simulink model "FOC_Motor_Control"  (R2020b)
settings: Solver=FixedStepDiscrete  StartTime=0.0  StopTime=10.0  FixedStep=Fixed_Step_Size  RelTol=1e-3
values from neighbouring files (symbols this model uses):
  Angle = 1.0    [Hall_Flux_FOC_Data.sldd]    (also in Motor_Control_Data.sldd)
  Cosine_table = 1.0 0.99999529 0.99999058 0.99998587 0.99998116 0.99996704 0.99995291 0.99993885 0.99992472 0.99990118 0.99987763 0.99985409 0.9998306 0.99979764 0.99976468 0.99973178 0.99969882 0.99965644 0.99961412 0.99957174 0.99952942 0.99947762 0.99942589 0.99937415 0.99932235 0.9992612 0.99920005 0.99913889 0.99907768 0.99900717 0.99893659 0.99886602 0.99879545 0.99871546 0.99863547 0.99855554 0.99847555 0.    [Hall_Flux_FOC_Data.sldd]    (also in Motor_Control_Data.sldd)
  Flux = 0.0109    [G474_FOC_LADRC.sldd]    (also in G474_FOC_NONOBSERVER.sldd = 0.0109
  HaLL_AngleShift = -0.25    [Hall_Flux_FOC_Data.sldd]
  HaLL_Sector1 = 5.236    [Hall_Flux_FOC_Data.sldd]
  HaLL_Sector2 = 1.0472    [Hall_Flux_FOC_Data.sldd]
  HaLL_Sector3 = 0.0    [Hall_Flux_FOC_Data.sldd]
  HaLL_Sector4 = 3.1415    [Hall_Flux_FOC_Data.sldd]
  HaLL_Sector5 = 4.1888    [Hall_Flux_FOC_Data.sldd]
  HaLL_Sector6 = 2.0944    [Hall_Flux_FOC_Data.sldd]
  HaLL_Timer_T = 1.0E-5    [Hall_Flux_FOC_Data.sldd]
  ID_Ki = 1.3    [Hall_Flux_FOC_Data.sldd]    (also in Motor_Control_Data.sldd = 48.0
  ID_Kp = 0.4    [Hall_Flux_FOC_Data.sldd]    (also in Motor_Control_Data.sldd = 0.84
  inverter = struct    [PMSM_Parameters.m]
  IQ_Ki = 1.6    [Hall_Flux_FOC_Data.sldd]    (also in Motor_Control_Data.sldd = 48.0
  IQ_Kp = 0.4    [Hall_Flux_FOC_Data.sldd]    (also in Motor_Control_Data.sldd = 1.869
  LADRC_b0 = 10000.0    [G474_FOC_LADRC.sldd]    (also in Hall_Flux_FOC_Data.sldd = 80000.0
  LADRC_Omega_c = 100.0    [G474_FOC_LADRC.sldd]    (also in Hall_Flux_FOC_Data.sldd = 80.0
  Ld = 0.0004    [Hall_Flux_FOC_Data.sldd]    (also in Motor_Control_Data.sldd = 0.00014
  Lq = 0.00045    [Hall_Flux_FOC_Data.sldd]    (also in Motor_Control_Data.sldd = 0.0003115
  OPL_Speed = 800.0    [Hall_Flux_FOC_Data.sldd]
  OPL_Time = 2.0    [Hall_Flux_FOC_Data.sldd]
  OPL_Torque = 3.0    [Hall_Flux_FOC_Data.sldd]
  Over_modulation = 0.0    [Hall_Flux_FOC_Data.sldd]    (also in Motor_Control_Data.sldd)
  pll_omega = 5000.0    [G474_FOC_LADRC.sldd]    (also in G474_FOC_NONOBSERVER.sldd)
  pll_xi = 10.0    [G474_FOC_LADRC.sldd]    (also in G474_FOC_NONOBSERVER.sldd)
  Pole_Pairs = 2.0    [Hall_Flux_FOC_Data.sldd]    (also in Motor_Control_Data.sldd = 4.0
  PWM_Frequency = 10000.0    [Hall_Flux_FOC_Data.sldd]    (also in Motor_Control_Data.sldd = 20000.0
  R = 0.405    [Hall_Flux_FOC_Data.sldd]    (also in Motor_Control_Data.sldd = 0.016
  Sine_table = 0.0 0.0015339879 0.0030679768 0.0046019657 0.0061359555 0.0076698866 0.0092038177 0.010737749 0.012271681 0.013805497 0.015339312 0.016873131 0.018406944 0.019940587 0.021474229 0.023007872 0.024541514 0.026074925 0.027608337 0.029141748 0.03067516 0.032208283 0.033741407 0.035274528 0.036807653 0.038340431 0.039873205 0.04140598 0.042938754 0.04447113 0.046003502 0.047535874 0.049068246 0.0506001    [Hall_Flux_FOC_Data.sldd]    (also in Motor_Control_Data.sldd)
  Speed_Ki = 0.06    [Hall_Flux_FOC_Data.sldd]    (also in Motor_Control_Data.sldd = 10.809
  Speed_Kp = 0.002    [Hall_Flux_FOC_Data.sldd]    (also in Motor_Control_Data.sldd = 0.08
  Speed_PI_OutputMax = 3.0    [Hall_Flux_FOC_Data.sldd]    (also in Motor_Control_Data.sldd = 700.0
  Speed_PI_OutputMin = -5.0    [Hall_Flux_FOC_Data.sldd]    (also in Motor_Control_Data.sldd = -700.0
  SpeedFilter_Fn = 0.3    [Hall_Flux_FOC_Data.sldd]    (also in Motor_Control_Data.sldd = 0.2
  TorqueMode = 0.0    [Hall_Flux_FOC_Data.sldd]    (also in Motor_Control_Data.sldd)
undefined symbols (not defined in the file or in its folder): DiscIntNeverNeededParam, Flux_Gain, Flux_Theta_Enable, magnitude, SVPWM
libraries: simulink x6, dspstat3 x1, pid_lib x1
(part 3 of 3)

== system FOC_Motor_Control/Motor_Control/Motor_Control_Function/Control_Command_2ms/Control_Command_2ms/Speed_PI/Speed_PI/Speed_Control ==
  Err : Inport
  Reset : Inport  Port=2
  Add : Sum
  Cons : Constant  Value=0  OutDataTypeStr=single
  Discrete-Time Integrator : DiscreteIntegrator  ExternalReset=level  SampleTime=-1  ICPrevOutput=DiscIntNeverNeededParam  ICPrevScaledInput=DiscIntNeverNeededParam
  Ki : Constant  Value=Speed_Ki  OutDataTypeStr=single
  Kp : Constant  Value=Speed_Kp  OutDataTypeStr=single
  Product : Product
  Product1 : Product
  Relational Operator1 : RelationalOperator  Operator===  OutDataTypeStr=boolean  RndMeth=Simplest
  Saturation : Saturate  UpperLimit=Speed_PI_OutputMax  LowerLimit=Speed_PI_OutputMin
  Scope : Scope
  Switch : Switch  Criteria=u2 > Threshold
  Unit Delay3 : UnitDelay  SampleTime=-1  HasFrameUpgradeWarning=on
  PI_Out : Outport
  wires:
  Kp/1 -> Product/1
  Err/1 -> Switch/1, Product/2
  Switch/1 -> Product1/2
  Product1/1 -> Discrete-Time Integrator/1
  Product/1 -> Add/1
  Add/1 -> Relational Operator1/1, Saturation/1
  Saturation/1 -> Relational Operator1/2, PI_Out/1
  Discrete-Time Integrator/1 -> Add/2, Scope/1
  Relational Operator1/1 -> Unit Delay3/1
  Ki/1 -> Product1/1
  Unit Delay3/1 -> Switch/2
  Cons/1 -> Switch/3
  Reset/1 -> Discrete-Time Integrator/2

== system FOC_Motor_Control/Motor_Control/Motor_Control_Function/FOC_Control_100us/FOC/D_Current_PI/ID_Control/Normal ==
  Bus_voltage : Inport
  Action Port : ActionPort  ActionPortLabel=elseif(u1==0)
  Gain : Gain  Gain=1/sqrt(3)
  Gain1 : Gain  Gain=-1/sqrt(3)
  Out1 : Outport
  Out2 : Outport  Port=2
  wires:
  Bus_voltage/1 -> Gain1/1, Gain/1
  Gain/1 -> Out1/1
  Gain1/1 -> Out2/1

== system FOC_Motor_Control/Motor_Control/Motor_Control_Function/FOC_Control_100us/FOC/D_Current_PI/ID_Control/Over_M ==
  Bus_voltage : Inport
  Action Port : ActionPort  ActionPortLabel=if(u1==1)
  Gain : Gain  Gain=2/3
  Gain1 : Gain  Gain=-2/3
  Out1 : Outport
  Out2 : Outport  Port=2
  wires:
  Bus_voltage/1 -> Gain1/1, Gain/1
  Gain/1 -> Out1/1
  Gain1/1 -> Out2/1

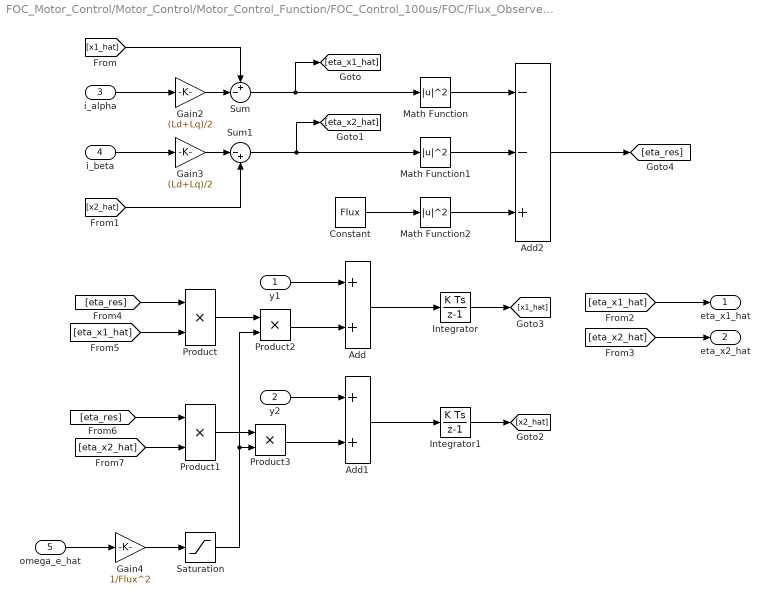
== system FOC_Motor_Control/Motor_Control/Motor_Control_Function/FOC_Control_100us/FOC/Flux_Observer/OBSERVER/Cacl_X1X2_Hat ==
  y1 : Inport  OutDataTypeStr=single
  y2 : Inport  Port=2  OutDataTypeStr=single
  i_alpha : Inport  Port=3  OutDataTypeStr=single
  i_beta : Inport  Port=4  OutDataTypeStr=single
  omega_e_hat : Inport  Port=5  OutDataTypeStr=single
  Add : Sum  OutDataTypeStr=single
  Add1 : Sum  OutDataTypeStr=single
  Add2 : Sum  Inputs=--+  OutDataTypeStr=single
  Constant : Constant  Value=Flux  OutDataTypeStr=single
  Gain2 : Gain  Gain=(Ld+Lq)/2  OutDataTypeStr=single
  Gain3 : Gain  Gain=(Ld+Lq)/2  OutDataTypeStr=single
  Gain4 : Gain  Gain=1/Flux^2  OutDataTypeStr=single
  Integrator : DiscreteIntegrator  SampleTime=-1  OutDataTypeStr=single  ICPrevOutput=DiscIntNeverNeededParam  ICPrevScaledInput=DiscIntNeverNeededParam  mask(DiscretizedDiscreteIntegrator){}
      mask init:
      | %zoh
  Integrator1 : DiscreteIntegrator  SampleTime=-1  OutDataTypeStr=single  ICPrevOutput=DiscIntNeverNeededParam  ICPrevScaledInput=DiscIntNeverNeededParam  mask(DiscretizedDiscreteIntegrator){}
      mask init:
      | %zoh
  Math Function : Math  Operator=magnitude^2  OutDataTypeStr=single  SaturateOnIntegerOverflow=on
  Math Function1 : Math  Operator=magnitude^2  OutDataTypeStr=single  SaturateOnIntegerOverflow=on
  Math Function2 : Math  Operator=magnitude^2  OutDataTypeStr=single  SaturateOnIntegerOverflow=on
  Product{,1..3} (4 alike) : Product  OutDataTypeStr=single
  Saturation : Saturate  UpperLimit=500e4  LowerLimit=20e4  OutDataTypeStr=single
  Sum : Sum  Inputs=+-|  OutDataTypeStr=single
  Sum1 : Sum  Inputs=|-+  OutDataTypeStr=single
  eta_x1_hat : Outport  OutDataTypeStr=single
  eta_x2_hat : Outport  Port=2  OutDataTypeStr=single
  wires:
  y1/1 -> Add/1
  Product3/1 -> Add1/2
  Product1/1 -> Product3/1
  Sum/1 -> [eta_x1_hat], Math Function/1
  Product/1 -> Product2/1
  Product2/1 -> Add/2
  Add/1 -> Integrator/1
  Add1/1 -> Integrator1/1
  Sum1/1 -> Math Function1/1, [eta_x2_hat]
  Integrator1/1 -> [x2_hat]
  y2/1 -> Add1/1
  Integrator/1 -> [x1_hat]
  i_beta/1 -> Gain3/1
  i_alpha/1 -> Gain2/1
  [x2_hat] -> Sum1/2
  Gain3/1 -> Sum1/1
  Math Function1/1 -> Add2/2
  Gain2/1 -> Sum/2
  [x1_hat] -> Sum/1
  Math Function/1 -> Add2/1
  Add2/1 -> [eta_res]
  [eta_x1_hat] -> eta_x1_hat/1
  [eta_x2_hat] -> eta_x2_hat/1
  [eta_res] -> Product/1
  [eta_x1_hat] -> Product/2
  [eta_res] -> Product1/1
  [eta_x2_hat] -> Product1/2
  Constant/1 -> Math Function2/1
  Math Function2/1 -> Add2/3
  omega_e_hat/1 -> Gain4/1
  Gain4/1 -> Saturation/1
  Saturation/1 -> Product2/2, Product3/2

== system FOC_Motor_Control/Motor_Control/Motor_Control_Function/FOC_Control_100us/FOC/Flux_Observer/OBSERVER/Cacl_Y1Y2 ==
  i_alpha : Inport  OutDataTypeStr=single
  u_alpha : Inport  Port=2  OutDataTypeStr=single
  i_beta : Inport  Port=3  OutDataTypeStr=single
  u_beta : Inport  Port=4  OutDataTypeStr=single
  omega_e_hat : Inport  Port=5  OutDataTypeStr=single
  Add4 : Sum  Inputs=-+  OutDataTypeStr=single
  Add5 : Sum  Inputs=-+  OutDataTypeStr=single
  Gain : Gain  Gain=0.005  OutDataTypeStr=single
  Gain1 : Gain  Gain=R  OutDataTypeStr=single
  Product : Product  OutDataTypeStr=single
  Product1 : Product  OutDataTypeStr=single
  Saturation : Saturate  UpperLimit=1  LowerLimit=0.8  OutDataTypeStr=single
  y1 : Outport  OutDataTypeStr=single
  y2 : Outport  Port=2  OutDataTypeStr=single
  wires:
  Add5/1 -> y2/1
  Product/1 -> Add4/1
  Product1/1 -> Add5/1
  u_beta/1 -> Add5/2
  i_beta/1 -> Product1/1
  Add4/1 -> y1/1
  i_alpha/1 -> Product/1
  u_alpha/1 -> Add4/2
  Gain/1 -> Saturation/1
  Saturation/1 -> Gain1/1
  omega_e_hat/1 -> Gain/1
  Gain1/1 -> Product/2, Product1/2

== system FOC_Motor_Control/Motor_Control/Motor_Control_Function/FOC_Control_100us/FOC/Flux_Observer/OBSERVER/LPF ==
  u : Inport
  Add : Sum  Inputs=+-
  Add1 : Sum
  Constant1 : Constant  Value=SpeedFilter_Fn  OutDataTypeStr=single
  Divide1 : Product  Inputs=**
  Unit Delay : UnitDelay  SampleTime=-1  HasFrameUpgradeWarning=on
  y : Outport
  wires:
  Constant1/1 -> Divide1/1
  u/1 -> Add/1
  Add/1 -> Divide1/2
  Divide1/1 -> Add1/1
  Unit Delay/1 -> Add/2, Add1/2
  Add1/1 -> Unit Delay/1, y/1

== system FOC_Motor_Control/Motor_Control/Motor_Control_Function/FOC_Control_100us/FOC/Flux_Observer/OBSERVER/PLL ==
  eta_x1_hat : Inport  OutDataTypeStr=single
  eta_x2_hat : Inport  Port=2  OutDataTypeStr=single
  Constant : Constant  Value=pll_omega  OutDataTypeStr=single  SampleTime=-1
  Discrete PID Controller : pid_lib/PID Controller  Controller=PI  Form=Parallel  TimeDomain=Discrete-time  UseExternalTs=off  SampleTime=-1  IntegratorMethod=Forward Euler  FilterMethod=Forward Euler  ControllerParametersSource=external  P=2*0.707*1650  I=1650*1650  D=0  UseFilter=on  N=100  TunerSelectOption=Transfer Function Based (PID Tuner App)  ZeroCross=off  InitialConditionSource=internal  InitialConditionForIntegrator=0  InitialConditionForFilter=0  DifferentiatorICPrevScaledInput=0  ExternalReset=none  TrackingMode=off  Kt=1  LimitOutput=on  SatLimitsSource=internal  UpperSaturationLimit=2500*2*pi*Pole_Pairs/60  LowerSaturationLimit=-2500*2*pi*Pole_Pairs/60  LinearizeAsGain=off  AntiWindupMode=clamping  Kb=1  POutMin=[]  POutMax=[]  IOutMin=[]  IOutMax=[]  DOutMin=[]  DOutMax=[]  NOutMin=[]  NOutMax=[]  SumOutMin=[]  SumOutMax=[]  SaturationOutMin=[]  SaturationOutMax=[]  PParamMin=[]  PParamMax=[]  IParamMin=[]  IParamMax=[]  DParamMin=[]  DParamMax=[]  NParamMin=[]  NParamMax=[]  KbParamMin=[]  KbParamMax=[]  KtParamMin=[]  KtParamMax=[]  KbOutMin=[]  KbOutMax=[]  KtOutMin=[]  KtOutMax=[]  IntegratorOutMin=[]  IntegratorOutMax=[]  FilterOutMin=[]  FilterOutMax=[]  SumI1OutMin=[]  SumI1OutMax=[]  SumI2OutMin=[]  SumI2OutMax=[]  SumI3OutMin=[]  SumI3OutMax=[]  SumI4OutMin=[]  SumI4OutMax=[]  SumDOutMin=[]  SumDOutMax=[]  DifferentiatorOutMin=[]  DifferentiatorOutMax=[]  FilterDiffOutCoefMin=[]  FilterDiffOutCoefMax=[]  ReciprocalOutMin=[]  ReciprocalOutMax=[]  SumDenOutMin=[]  SumDenOutMax=[]  SumNumOutMin=[]  SumNumOutMax=[]  DivideOutMin=[]  DivideOutMax=[]  UdiffTsProdOutMin=[]  UdiffTsProdOutMax=[]  NTsProdOutMin=[]  NTsProdOutMax=[]  UintegralTsProdOutMin=[]  UintegralTsProdOutMax=[]  UngainTsProdOutMin=[]  UngainTsProdOutMax=[]  IntegratorContinuousStateAttributes=''  IntegratorStateMustResolveToSignalObject=off  IntegratorRTWStateStorageClass=Auto  FilterContinuousStateAttributes=''  FilterStateMustResolveToSignalObject=off  FilterRTWStateStorageClass=Auto  ParallelPVariant=ExternalParameters  IdealPVariant=Disabled  IVariant=ExternalParameters  DVariant=Disabled  IntegratorVariant=Discrete  SatVariant=Enabled  AWVariant=DiscClampingParallel  PCopyVariant=Disabled  TRVariant=Disabled  FdbkBlocksVariant=Forward  IdealPFdbkVariant=Disabled  SatFdbkVariant=Disabled  DerivativeFilterVariant=Disabled  NVariant=Disabled  NCopyVariant=Disabled_SignalSpec  FilterICVariant=Disabled  IntegratorICVariant=InternalICs  ExternalResetVariant=Disabled  TRSumVariant=Passthrough  SumFdbkVariant=Disabled  SumVariant=Sum_PI  TsampFilterVariant=InternalTs  TsampNgainVariant=Passthrough  TsampIntegralVariant=Passthrough  ExternalSaturationOutDataTypeStr=Inherit: Same as second input
  Gain : Gain  Gain=pll_xi  OutDataTypeStr=single
  Product : Product  OutDataTypeStr=single
  Product1 : Product  OutDataTypeStr=single
  Product2 : Product  OutDataTypeStr=single
  Scope : Scope  NumInputPorts=2
  Sine_Cosine : Subsystem  TreatAsAtomicUnit=on
      settings: RTWSystemCode=Nonreusable function  RTWFcnNameOpts=Use subsystem name
  Sum : Sum  Inputs=-|+  OutDataTypeStr=single
  integrator : Subsystem
  Obs_Theta : Outport  OutDataTypeStr=single
  omega_e_hat : Outport  Port=2  OutDataTypeStr=single
  wires:
  Product/1 -> Sum/1
  Product1/1 -> Sum/2
  Sum/1 -> Discrete PID Controller/1
  Sine_Cosine/2(Cos) -> Product1/2
  Sine_Cosine/1(Sin) -> Product/1
  integrator/1(y(k-1)) -> Sine_Cosine/1(P), Obs_Theta/1  "ObserverTheta"
  eta_x1_hat/1 -> Scope/1, Product/2
  eta_x2_hat/1 -> Scope/2, Product1/1
  Gain/1 -> Discrete PID Controller/2
  Constant/1 -> Product2/2, Product2/1, Gain/1
  Product2/1 -> Discrete PID Controller/3
  Discrete PID Controller/1 -> omega_e_hat/1, integrator/1(x(k))  "Obs_We"

== system FOC_Motor_Control/Motor_Control/Motor_Control_Function/FOC_Control_100us/FOC/Q_Current_PI/IQ_Control/Normal ==
  Bus_voltage : Inport
  Action Port : ActionPort  ActionPortLabel=elseif(u1==0)
  Gain : Gain  Gain=1/sqrt(3)
  Gain1 : Gain  Gain=-1/sqrt(3)
  Out1 : Outport
  Out2 : Outport  Port=2
  wires:
  Bus_voltage/1 -> Gain1/1, Gain/1
  Gain/1 -> Out1/1
  Gain1/1 -> Out2/1

== system FOC_Motor_Control/Motor_Control/Motor_Control_Function/FOC_Control_100us/FOC/Q_Current_PI/IQ_Control/Over_M ==
  Bus_voltage : Inport
  Action Port : ActionPort  ActionPortLabel=if(u1==1)
  Gain : Gain  Gain=2/3
  Gain1 : Gain  Gain=-2/3
  Out1 : Outport
  Out2 : Outport  Port=2
  wires:
  Bus_voltage/1 -> Gain1/1, Gain/1
  Gain/1 -> Out1/1
  Gain1/1 -> Out2/1

== system FOC_Motor_Control/Motor_Control/Motor_Control_Function/FOC_Control_100us/FOC/Flux_Observer/OBSERVER/PLL/Sine_Cosine ==
  note: Sine Cosine Coefficients
  P : Inport
  Cosine : Lookup_n-D  NumberOfTableDimensions=1  LookupTableObject=''  BreakpointsForDimension1=[0:2*pi/4095:2*pi]  BreakpointsForDimension1FirstPoint=10  BreakpointsForDimension2FirstPoint=10  BreakpointsForDimension1Spacing=12  BreakpointsForDimension2Spacing=12  IndexSearchMethod=Evenly spaced points  Table=Cosine_table  InterpMethod=Flat  DiagnosticForOutOfRangeInput=Error  InternalRulePriority=Speed  RndMeth=Simplest  InputSameDT=on
  Saturation : Saturate  UpperLimit=2*pi-0.001  LowerLimit=0+0.001
  Scope : Scope  NumInputPorts=2
  Sine : Lookup_n-D  NumberOfTableDimensions=1  LookupTableObject=''  BreakpointsForDimension1=[0:2*pi/4095:2*pi]  BreakpointsForDimension1FirstPoint=10  BreakpointsForDimension2FirstPoint=10  BreakpointsForDimension1Spacing=12  BreakpointsForDimension2Spacing=12  IndexSearchMethod=Evenly spaced points  Table=Sine_table  InterpMethod=Flat  DiagnosticForOutOfRangeInput=Error  InternalRulePriority=Speed  RndMeth=Simplest  InputSameDT=on
  Sin : Outport  VectorParamsAs1DForOutWhenUnconnected=off
  Cos : Outport  Port=2  VectorParamsAs1DForOutWhenUnconnected=off
  wires:
  P/1 -> Saturation/1  "position"
  Sine/1 -> Scope/1, Sin/1
  Cosine/1 -> Scope/2, Cos/1
  Saturation/1 -> Cosine/1, Sine/1

== system FOC_Motor_Control/Motor_Control/Motor_Control_Function/FOC_Control_100us/FOC/Flux_Observer/OBSERVER/PLL/integrator ==
  x(k) : Inport  OutDataTypeStr=single
  RangeLimit : Subsystem
  Sum1 : Sum  Inputs=|++  OutDataTypeStr=single
  Ts : Gain  Gain=1/PWM_Frequency  OutDataTypeStr=single
  Unit Delay : UnitDelay  SampleTime=-1  HasFrameUpgradeWarning=on
  y(k-1) : Outport  OutDataTypeStr=single
  wires:
  x(k)/1 -> Ts/1
  Ts/1 -> Sum1/1
  Sum1/1 -> RangeLimit/1(In)  "y(k)"
  Unit Delay/1 -> y(k-1)/1, Sum1/2
  RangeLimit/1(Theta) -> Unit Delay/1

== system FOC_Motor_Control/Motor_Control/Motor_Control_Function/FOC_Control_100us/FOC/Flux_Observer/OBSERVER/PLL/integrator/RangeLimit ==
  In : Inport  OutDataTypeStr=single
  Constant : Constant  Value=2*pi  OutDataTypeStr=single  SampleTime=-1
  Constant1 : Constant  Value=0  OutDataTypeStr=single  SampleTime=-1
  If : If  NumInputs=2  IfExpression=u1  ElseIfExpressions=u2
  If Action Subsystem : Subsystem  TreatAsAtomicUnit=on
  If Action Subsystem1 : Subsystem  TreatAsAtomicUnit=on
  If Action Subsystem2 : Subsystem  TreatAsAtomicUnit=on
  Merge : Merge  Inputs=3
  Relational Operator : RelationalOperator  Operator=>  OutDataTypeStr=boolean  RndMeth=Simplest
  Relational Operator1 : RelationalOperator  Operator=<  OutDataTypeStr=boolean  RndMeth=Simplest
  Theta : Outport  OutDataTypeStr=single
  wires:
  Relational Operator/1 -> If/1
  Constant/1 -> Relational Operator/2
  Constant1/1 -> Relational Operator1/2
  In/1 -> Relational Operator1/1, If Action Subsystem2/1(In1), If Action Subsystem1/1(In1), If Action Subsystem/1(In1), Relational Operator/1
  Relational Operator1/1 -> If/2
  Merge/1 -> Theta/1
  If/3 -> If Action Subsystem2/Action
  If/2 -> If Action Subsystem/Action
  If/1 -> If Action Subsystem1/Action
  If Action Subsystem2/1(Out1) -> Merge/1
  If Action Subsystem/1(Out1) -> Merge/2
  If Action Subsystem1/1(Out1) -> Merge/3

== system FOC_Motor_Control/Motor_Control/Motor_Control_Function/FOC_Control_100us/FOC/Flux_Observer/OBSERVER/PLL/integrator/RangeLimit/If Action Subsystem ==
  In1 : Inport  OutDataTypeStr=single
  Action Port : ActionPort  ActionPortLabel=elseif(u2)
  Constant : Constant  Value=2*pi  OutDataTypeStr=single  SampleTime=-1
  Sum : Sum  Inputs=|++  OutDataTypeStr=single
  Out1 : Outport  OutDataTypeStr=single
  wires:
  In1/1 -> Sum/1
  Constant/1 -> Sum/2
  Sum/1 -> Out1/1

== system FOC_Motor_Control/Motor_Control/Motor_Control_Function/FOC_Control_100us/FOC/Flux_Observer/OBSERVER/PLL/integrator/RangeLimit/If Action Subsystem1 ==
  In1 : Inport  OutDataTypeStr=single
  Action Port : ActionPort  ActionPortLabel=if(u1)
  Constant : Constant  Value=2*pi  OutDataTypeStr=single  SampleTime=-1
  Sum : Sum  Inputs=|+-  OutDataTypeStr=single
  Out1 : Outport  OutDataTypeStr=single
  wires:
  In1/1 -> Sum/1
  Constant/1 -> Sum/2
  Sum/1 -> Out1/1

== system FOC_Motor_Control/Motor_Control/Motor_Control_Function/FOC_Control_100us/FOC/Flux_Observer/OBSERVER/PLL/integrator/RangeLimit/If Action Subsystem2 ==
  In1 : Inport  OutDataTypeStr=single
  Action Port : ActionPort  ActionPortLabel=else
  Out1 : Outport  OutDataTypeStr=single
  wires:
  In1/1 -> Out1/1

== stateflow chart FOC_Motor_Control/Motor_Control/Motor_Control_Function/FOC_Control_100us/FOC/Chart ==
  state OPL
    en,du:
    Motor_State=1;
  state Standby
    en,du:
    Motor_State=0;
  state CLP
    en,du:
    Motor_State=2;
  (default) -> Standby
  Standby -> OPL : [OLP_Enable==1 & Motor_Start==0]
  OPL -> CLP [order 1] : [Motor_Start==0 & after(OPL_Time,sec) & Measure_Speed>500 ]
  OPL -> Standby [order 2] : [OLP_Enable==0 & Motor_Start==1]
  CLP -> Standby : [OLP_Enable==0 & Motor_Start==1]
  data: Measure_Speed input single; Motor_State output uint8; OLP_Enable input uint8; Motor_Start input uint8; OPL_Time input single
